simulink model "Automatic_Control2_345"  (R2021a)
settings: Solver=VariableStepAuto  StartTime=0.0  StopTime=5  RelTol=1e-3
values from neighbouring files (symbols this model uses):
  b = 0.006    [Automatic_Control2.m]
  b_high = 0.0066    [Automatic_Control2.m]
  b_low = 0.0054    [Automatic_Control2.m]
  Jm = 0.05    [Automatic_Control2.m]
  Jm_high = 0.055    [Automatic_Control2.m]
  Jm_low = 0.045    [Automatic_Control2.m]
  Ke = 0.05    [Automatic_Control2.m]
  Ke_high = 0.055    [Automatic_Control2.m]
  Ke_low = 0.045    [Automatic_Control2.m]
  Kt = 0.05    [Automatic_Control2.m]
  Kt_high = 0.055    [Automatic_Control2.m]
  Kt_low = 0.045    [Automatic_Control2.m]
  La = 0.01    [Automatic_Control2.m]
  La_high = 0.011    [Automatic_Control2.m]
  La_low = 0.009    [Automatic_Control2.m]
  Ra = 10    [Automatic_Control2.m]
  Ra_high = 11.0    (= 11)    [Automatic_Control2.m]
  Ra_low = 9.0    (= 9)    [Automatic_Control2.m]
undefined symbols (not defined in the file or in its folder): sigbuilder_block
libraries: simulink x2
settings Model: Creator=Rosa  LastModifiedBy=han_jjun_mac
settings SolverCC: AlgebraicLoopSolver=TrustRegion
settings DebuggingCC: SFMachineParentedDataDiag=warning

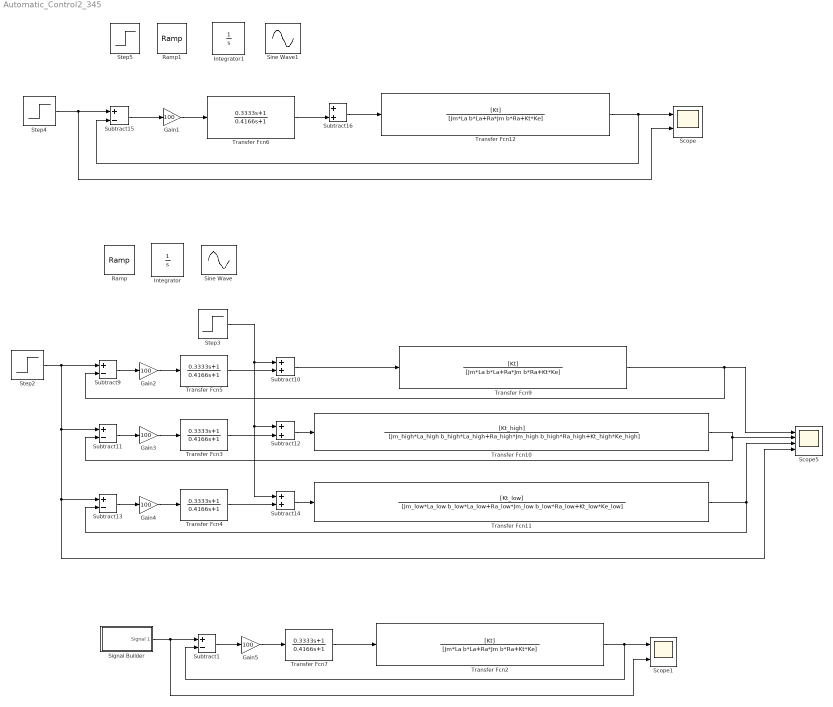
== system Automatic_Control2_345 ==
  Gain{1..5} (5 alike) : Gain  Gain=100
  Integrator : Integrator
  Integrator1 : Integrator
  Ramp : simulink/Sources/Ramp  slope=1  start=0  InitialOutput=0
  Ramp1 : simulink/Sources/Ramp  slope=1  start=0  InitialOutput=0
  Scope : Scope  NumInputPorts=2
  Scope1 : Scope  NumInputPorts=2
  Scope5 : Scope  NumInputPorts=4
  Signal Builder : Subsystem  Tag=STV Subsys  LoadFcn=sigbuilder_block('load');  StartFcn=sigbuilder_block('start');  StopFcn=sigbuilder_block('stop');  ClipboardFcn=sigbuilder_block('clipboard');  mask(Sigbuilder block){tuvar=[0:10]}
      mask help: Simulink:masks:SigbuilderBlock_MD
      mask init:
      | if ~strcmp(get_param(bdroot(gcbh),'SimulationStatus'),'stopped') tuvar = sigbuilder_block('maskInit'); end
      settings: CopyFcn=sigbuilder_block('copy');  DeleteFcn=sigbuilder_block('delete');  ModelCloseFcn=sigbuilder_block('modelClose');  PreSaveFcn=sigbuilder_block('preSave');  PauseFcn=sigbuilder_block('pause');  ContinueFcn=sigbuilder_block('continue');  NameChangeFcn=sigbuilder_block('namechange');  OpenFcn=sigbuilder_block('open',[278.4 116.4 531 400.2 ]);  CloseFcn=sigbuilder_block('close');
      mask Display: plot(0, 0, 100, 100,[2, 2, 32, 32, 2], [68, 8, 8, 68, 68],[32, 2], [38, 38], [32, 19, 2],[53, 60, 44], [32, 17, 17, 2],[16, 16, 31, 31]);txt = getActiveGroup(gcbh);text(2, 100, txt,'verticalAlignment', 'top');
  Sine Wave : Sin  SampleTime=0
  Sine Wave1 : Sin  SampleTime=0
  Step2 : Step  Time=0  SampleTime=0
  Step3 : Step  Time=0  SampleTime=0
  Step4 : Step  Time=0  SampleTime=0
  Step5 : Step  Time=0  After=2  SampleTime=0
  Subtract{1,9,11,13,15} (5 alike) : Sum  Inputs=+-
  Subtract{10,12,14,16} (4 alike) : Sum
  Transfer Fcn10 : TransferFcn  Numerator=[Kt_high]  Denominator=[Jm_high*La_high b_high*La_high+Ra_high*Jm_high b_high*Ra_high+Kt_high*Ke_high]
  Transfer Fcn11 : TransferFcn  Numerator=[Kt_low]  Denominator=[Jm_low*La_low b_low*La_low+Ra_low*Jm_low b_low*Ra_low+Kt_low*Ke_low]
  Transfer Fcn12 : TransferFcn  Numerator=[Kt]  Denominator=[Jm*La b*La+Ra*Jm b*Ra+Kt*Ke]
  Transfer Fcn2 : TransferFcn  Numerator=[Kt]  Denominator=[Jm*La b*La+Ra*Jm b*Ra+Kt*Ke]
  Transfer Fcn{3..7} (5 alike) : TransferFcn  Numerator=[0.3333 1]  Denominator=[0.4166 1]
  Transfer Fcn9 : TransferFcn  Numerator=[Kt]  Denominator=[Jm*La b*La+Ra*Jm b*Ra+Kt*Ke]
  wires:
  Transfer Fcn2/1 -> Scope1/1, Subtract1/2
  Signal Builder/1(Signal 1) -> Scope1/2, Subtract1/1
  Subtract16/1 -> Transfer Fcn12/1
  Transfer Fcn12/1 -> Subtract15/2, Scope/1
  Step4/1 -> Scope/2, Subtract15/1
  Step2/1 -> Subtract9/1, Subtract11/1, Subtract13/1, Scope5/4
  Subtract10/1 -> Transfer Fcn9/1
  Subtract12/1 -> Transfer Fcn10/1
  Transfer Fcn9/1 -> Subtract9/2, Scope5/1
  Transfer Fcn10/1 -> Subtract11/2, Scope5/2
  Transfer Fcn11/1 -> Subtract13/2, Scope5/3
  Subtract14/1 -> Transfer Fcn11/1
  Subtract15/1 -> Gain1/1
  Gain1/1 -> Transfer Fcn6/1
  Transfer Fcn6/1 -> Subtract16/2
  Subtract9/1 -> Gain2/1
  Transfer Fcn5/1 -> Subtract10/2
  Gain3/1 -> Transfer Fcn3/1
  Subtract11/1 -> Gain3/1
  Transfer Fcn3/1 -> Subtract12/2
  Gain4/1 -> Transfer Fcn4/1
  Subtract13/1 -> Gain4/1
  Transfer Fcn4/1 -> Subtract14/2
  Step3/1 -> Subtract14/1, Subtract12/1, Subtract10/1
  Gain5/1 -> Transfer Fcn7/1
  Subtract1/1 -> Gain5/1
  Transfer Fcn7/1 -> Transfer Fcn2/1
  Gain2/1 -> Transfer Fcn5/1

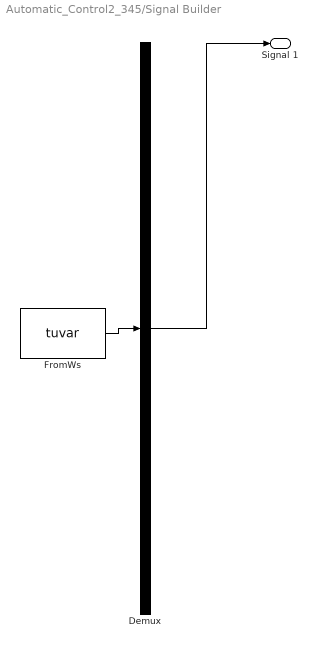
== system Automatic_Control2_345/Signal Builder ==
  Demux : Demux  Tag=STV Demux  Outputs=1
      settings: DisplayOption=none
  FromWs : FromWorkspace  Tag=STV FromWs  VariableName=tuvar
      SigBuilderData=|
      | common.afterFinalStr = 'Extrapolate'
      | common.sampleTime = 0
      | dataSet.timeRange = [0 15]
      | dataSet.name = 'Group 1'
      | sbobj.Groups.Name = 'Group 1'
      | sbobj.Groups.Signals.Name = 'Signal 1'
      | sbobj.Groups.Signals.XData = [0 1 2 10 15]
      | sbobj.Groups.Signals.YData = [0 100 100 0 0]
      | sbobj.Groups.TimeRange = [0 15]
  Signal 1 : Outport  Tag=STV Outport
  wires:
  Demux/1 -> Signal 1/1
  FromWs/1 -> Demux/1
